simulink model "PBR_PI"  (R2021b)
settings: Solver=VariableStepAuto  StartTime=0.0  StopTime=500  RelTol=1e-3
values from neighbouring files (symbols this model uses):
  b = 0.0008    [PBR_estim_5_param.m]    (also in PBR_optim_orizont.m)
  Ea = 200    [PBR_estim_5_param.m]    (also in PBR_optim_orizont.m)
  Es = 870    [PBR_estim_5_param.m]    (also in PBR_optim_orizont.m)
  I0 = 500    [PBR_estim_5_param.m]    (also in PBR_optim_orizont.m)
  Kn = params(3)    [PBR_estim_5_param.m]    (also in PBR_optim_orizont.m = 0.13236)
  Ks = params(2)    [PBR_estim_5_param.m]    (also in PBR_optim_orizont.m = 101.2637)
  L = 0.054    [PBR_estim_5_param.m]    (also in PBR_optim_orizont.m)
  mud = params(5)    [PBR_estim_5_param.m]    (also in PBR_optim_orizont.m = 0.010177)
  mumax = params(1)    [PBR_estim_5_param.m]    (also in PBR_optim_orizont.m = 0.21692)
  N0 = 2    [PBR_estim_5_param.m]    (also in PBR_optim_orizont.m = 1.5)
  Nin = 1    [PBR_estim_5_param.m]    (also in PBR_optim_orizont.m = 2)
  X0 = 0.1    [PBR_estim_5_param.m]    (also in PBR_optim_orizont.m)
  Ynx = params(4)    [PBR_estim_5_param.m]    (also in PBR_optim_orizont.m = 0.043508)
libraries: slpidlib x1
settings Model: Creator=georg
settings SolverCC: AlgebraicLoopSolver=TrustRegion
settings DataIOCC: ReturnWorkspaceOutputs=off
settings DebuggingCC: ArithmeticOperatorsInVariantConditions=warning
settings SFSimCC: CustomCodeUndefinedFunction=UseInterfaceOnly
settings RTWCC: DLArmComputeVersion=20.02.1

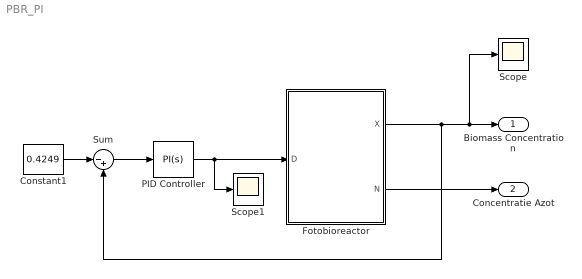
== system PBR_PI ==
  Constant1 : Constant  Value=0.4249
  Fotobioreactor : Subsystem
  PID Controller : slpidlib/PID Controller  Controller=PI  Form=Parallel  TimeDomain=Continuous-time  UseExternalTs=off  SampleTime=-1  IntegratorMethod=Forward Euler  FilterMethod=Forward Euler  ControllerParametersSource=internal  P=8  I=0.01  D=0  N=100  UseFilter=on  TunerSelectOption=Transfer Function Based (PID Tuner App)  InitialConditionSource=internal  InitialConditionForIntegrator=0  InitialConditionForFilter=0  DifferentiatorICPrevScaledInput=0  ExternalReset=none  TrackingMode=off  Kt=1  LimitOutput=on  SatLimitsSource=internal  UpperSaturationLimit=inf  LowerSaturationLimit=0  LinearizeAsGain=on  AntiWindupMode=none  Kb=1  POutMin=[]  POutMax=[]  IOutMin=[]  IOutMax=[]  DOutMin=[]  DOutMax=[]  NOutMin=[]  NOutMax=[]  SumOutMin=[]  SumOutMax=[]  SaturationOutMin=[]  SaturationOutMax=[]  PParamMin=[]  PParamMax=[]  IParamMin=[]  IParamMax=[]  DParamMin=[]  DParamMax=[]  NParamMin=[]  NParamMax=[]  KbParamMin=[]  KbParamMax=[]  KtParamMin=[]  KtParamMax=[]  KbOutMin=[]  KbOutMax=[]  KtOutMin=[]  KtOutMax=[]  IntegratorOutMin=[]  IntegratorOutMax=[]  FilterOutMin=[]  FilterOutMax=[]  SumI1OutMin=[]  SumI1OutMax=[]  SumI2OutMin=[]  SumI2OutMax=[]  SumI3OutMin=[]  SumI3OutMax=[]  SumI4OutMin=[]  SumI4OutMax=[]  SumDOutMin=[]  SumDOutMax=[]  DifferentiatorOutMin=[]  DifferentiatorOutMax=[]  FilterDiffOutCoefMin=[]  FilterDiffOutCoefMax=[]  ReciprocalOutMin=[]  ReciprocalOutMax=[]  SumDenOutMin=[]  SumDenOutMax=[]  SumNumOutMin=[]  SumNumOutMax=[]  DivideOutMin=[]  DivideOutMax=[]  UdiffTsProdOutMin=[]  UdiffTsProdOutMax=[]  NTsProdOutMin=[]  NTsProdOutMax=[]  UintegralTsProdOutMin=[]  UintegralTsProdOutMax=[]  UngainTsProdOutMin=[]  UngainTsProdOutMax=[]  IntegratorContinuousStateAttributes=''  IntegratorStateMustResolveToSignalObject=off  IntegratorRTWStateStorageClass=Auto  FilterContinuousStateAttributes=''  FilterStateMustResolveToSignalObject=off  FilterRTWStateStorageClass=Auto  ParallelPVariant=InternalParameters  IdealPVariant=Disabled  IVariant=InternalParameters  DVariant=Disabled  IntegratorVariant=Continuous  SatVariant=Enabled  AWVariant=Passthrough  PCopyVariant=Disabled  TRVariant=Disabled  FdbkBlocksVariant=Forward  IdealPFdbkVariant=Disabled  SatFdbkVariant=Disabled  DerivativeFilterVariant=Disabled  NVariant=Disabled  NCopyVariant=Disabled_SignalSpec  FilterICVariant=Disabled  IntegratorICVariant=InternalICs  ExternalResetVariant=Disabled  TRSumVariant=Passthrough  SumFdbkVariant=Disabled  SumVariant=Sum_PI  TsampFilterVariant=InternalTs  TsampNgainVariant=Passthrough  TsampIntegralVariant=Disabled_SignalSpec  ExternalSaturationOutDataTypeStr=Inherit: Same as second input
  Scope : Scope
  Scope1 : Scope
  Sum : Sum  Inputs=|-+
  Biomass Concentration : Outport
  Concentratie Azot : Outport  Port=2
  wires:
  Fotobioreactor/1(X) -> Sum/2, Scope/1, Biomass Concentration/1
  Fotobioreactor/2(N) -> Concentratie Azot/1
  PID Controller/1 -> Fotobioreactor/1(D), Scope1/1
  Constant1/1 -> Sum/1
  Sum/1 -> PID Controller/1

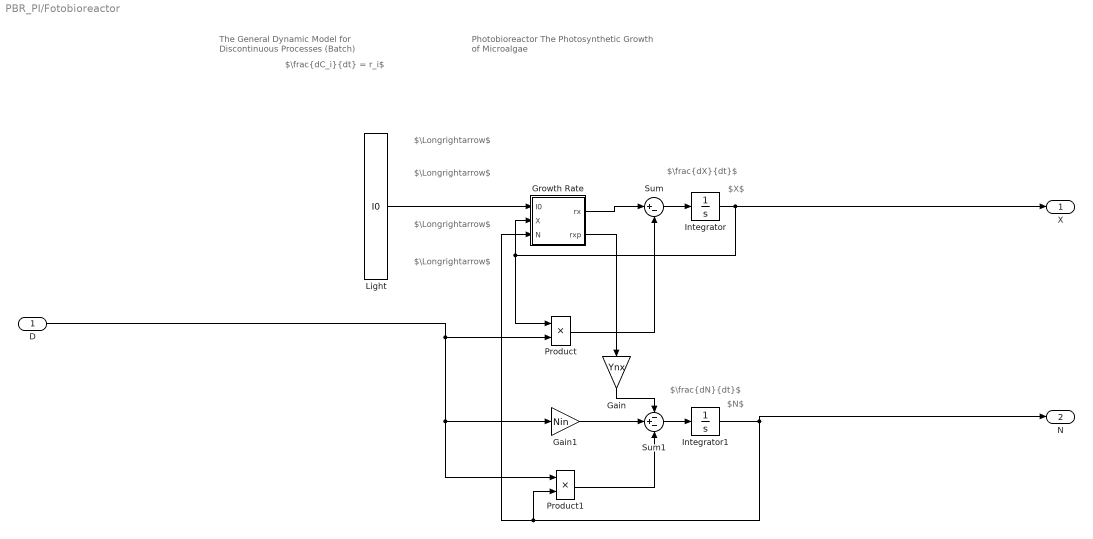
== system PBR_PI/Fotobioreactor ==
  note: The General Dynamic Model for
      | Discontinuous Processes (Batch)
  note: Photobioreactor
      | The Photosynthetic Growth of Microalgae
  note: $\Longrightarrow$
  note: $\frac{dC_i}{dt} = r_i$
  note: $\Longrightarrow$
  note: $\Longrightarrow$
  note: $\Longrightarrow$
  note: $\frac{dX}{dt}$
  note: $X$
  note: $\frac{dN}{dt}$
  note: $N$
  D : Inport
  Gain : Gain  Gain=Ynx
  Gain1 : Gain  Gain=Nin
  Growth Rate : Subsystem
  Integrator : Integrator  InitialCondition=X0
  Integrator1 : Integrator  InitialCondition=N0
  Light : Constant  Value=I0
  Product : Product
  Product1 : Product
  Sum : Sum  Inputs=|+-
  Sum1 : Sum  Inputs=-+-
  X : Outport
  N : Outport  Port=2
  wires:
  Gain1/1 -> Sum1/2
  Growth Rate/2(rxp) -> Gain/1
  Sum1/1 -> Integrator1/1
  Product1/1 -> Sum1/3
  Light/1 -> Growth Rate/1(I0)
  Product/1 -> Sum/2
  Gain/1 -> Sum1/1
  D/1 -> Product1/1, Gain1/1, Product/2
  Sum/1 -> Integrator/1
  Growth Rate/1(rx) -> Sum/1
  Integrator/1 -> X/1, Product/1, Growth Rate/2(X)
  Integrator1/1 -> N/1, Product1/2, Growth Rate/3(N)

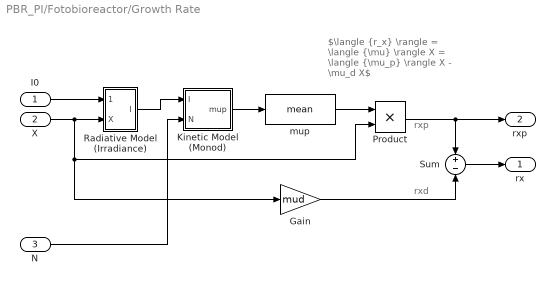
== system PBR_PI/Fotobioreactor/Growth Rate ==
  note: $\langle {r_x} \rangle = \langle {\mu} \rangle X = \langle {\mu_p} \rangle X - \mu_d X$
  note: rxd
  note: rxp
  I0 : Inport
  X : Inport  Port=2
  N : Inport  Port=3
  Gain : Gain  Gain=mud
  Kinetic Model (Monod) : Subsystem
  Product : Product
  Radiative Model (Irradiance) : Subsystem
  Sum : Sum  Inputs=+-
  mup : MATLABFcn  MATLABFcn=mean
  rx : Outport  VectorParamsAs1DForOutWhenUnconnected=off
  rxp : Outport  Port=2  VectorParamsAs1DForOutWhenUnconnected=off
  wires:
  X/1 -> Product/2, Gain/1, Radiative Model (Irradiance)/2(X)
  Gain/1 -> Sum/2
  Sum/1 -> rx/1
  I0/1 -> Radiative Model (Irradiance)/1(I0)
  Kinetic Model (Monod)/1(mup) -> mup/1
  Radiative Model (Irradiance)/1(I) -> Kinetic Model (Monod)/1(I)
  mup/1 -> Product/1
  Product/1 -> Sum/1, rxp/1
  N/1 -> Kinetic Model (Monod)/2(N)

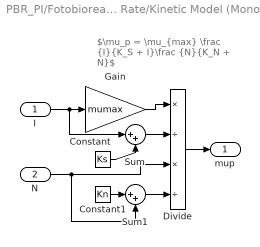
== system PBR_PI/Fotobioreactor/Growth Rate/Kinetic Model (Monod) ==
  note: $\mu_p = \mu_{max} \frac {I}{K_S + I}\frac {N}{K_N + N}$
  I : Inport
  N : Inport  Port=2
  Constant : Constant  Value=Ks
  Constant1 : Constant  Value=Kn
  Divide : Product  Inputs=*/*/
  Gain : Gain  Gain=mumax
  Sum : Sum  Inputs=|++
  Sum1 : Sum  Inputs=|++
  mup : Outport  VectorParamsAs1DForOutWhenUnconnected=off
  wires:
  Constant/1 -> Sum/2
  Sum/1 -> Divide/2
  I/1 -> Gain/1, Sum/1
  Gain/1 -> Divide/1
  Divide/1 -> mup/1
  N/1 -> Sum1/2, Divide/3
  Sum1/1 -> Divide/4
  Constant1/1 -> Sum1/1

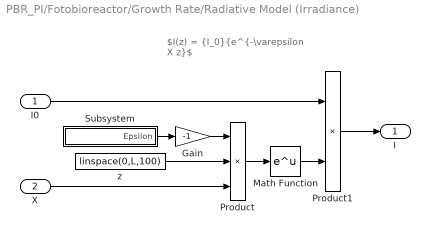
== system PBR_PI/Fotobioreactor/Growth Rate/Radiative Model (Irradiance) ==
  note: $I(z) = {I_0}{e^{-\varepsilon X z}$
  I0 : Inport
  X : Inport  Port=2
  Gain : Gain  Gain=-1
  Math Function : Math  SignedPower=on  SaturateOnIntegerOverflow=on
  Product : Product  Inputs=3
  Product1 : Product
  Subsystem : Subsystem
  z : Constant  Value=linspace(0,L,100)
  I : Outport  VectorParamsAs1DForOutWhenUnconnected=off
  wires:
  Gain/1 -> Product/1
  Subsystem/1(Epsilon) -> Gain/1
  I0/1 -> Product1/1
  z/1 -> Product/2
  X/1 -> Product/3
  Math Function/1 -> Product1/2
  Product1/1 -> I/1
  Product/1 -> Math Function/1

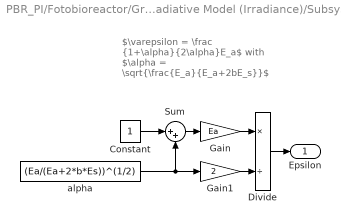
== system PBR_PI/Fotobioreactor/Growth Rate/Radiative Model (Irradiance)/Subsystem ==
  note: $\varepsilon = \frac {1+\alpha}{2\alpha}E_a$ with $\alpha = \sqrt{\frac{E_a}{E_a+2bE_s}}$
  Constant : Constant
  Divide : Product  Inputs=*/
  Gain : Gain  Gain=Ea
  Gain1 : Gain  Gain=2
  Sum : Sum  Inputs=|++
  alpha : Constant  Value=(Ea/(Ea+2*b*Es))^(1/2)
  Epsilon : Outport  VectorParamsAs1DForOutWhenUnconnected=off
  wires:
  Gain1/1 -> Divide/2
  Constant/1 -> Sum/1
  Sum/1 -> Gain/1
  alpha/1 -> Sum/2, Gain1/1
  Gain/1 -> Divide/1
  Divide/1 -> Epsilon/1
